simulink model "Pendulum_Controller"  (R2023a)
settings: Solver=ode4  StartTime=0.0  StopTime=5  FixedStep=0.001  RelTol=1e-3
settings Model: Creator=Fasih  LastModifiedBy=Fasih

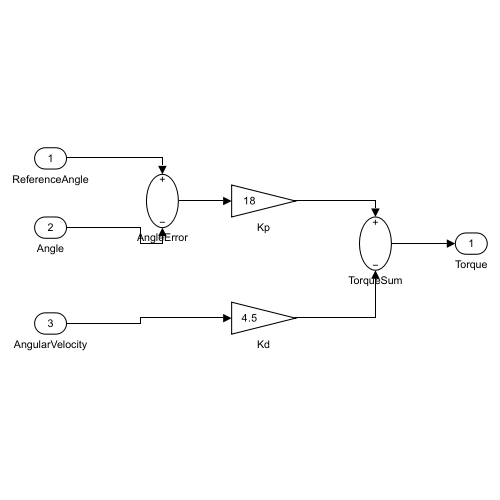
[thumbnail: Simulink's stored preview of the top-level diagram]
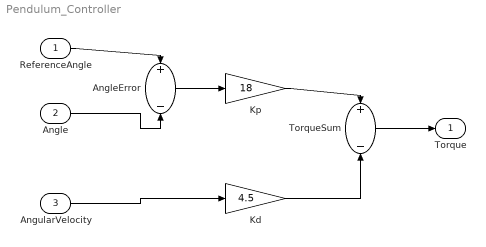
== system Pendulum_Controller ==
  ReferenceAngle : Inport
  Angle : Inport  Port=2
  AngularVelocity : Inport  Port=3
  AngleError : Sum  Inputs=+-
  Kd : Gain  Gain=4.5
  Kp : Gain  Gain=18
  TorqueSum : Sum  Inputs=+-
  Torque : Outport
  wires:
  ReferenceAngle/1 -> AngleError/1
  Angle/1 -> AngleError/2
  AngleError/1 -> Kp/1
  AngularVelocity/1 -> Kd/1
  Kp/1 -> TorqueSum/1
  Kd/1 -> TorqueSum/2
  TorqueSum/1 -> Torque/1
